simulink model "plltrans"  (R2017a)
settings: Solver=FixedStepAuto  StartTime=0.0  StopTime=150E-6  RelTol=1e-3
libraries: cstblocks x2, simulink x1, hdlsllib x1
settings Model: Creator=fritz  LastModifiedBy=beckmanf
settings OptimizationCC: BlockReduction=off  ConditionallyExecuteInputs=off  DefaultParameterBehavior=Inlined
settings DebuggingCC: AlgebraicLoopMsg=error  SingleTaskRateTransMsg=error
settings HardwareCC: ProdBitPerPointer=32  ProdBitPerSizeT=32  ProdBitPerPtrDiffT=32  ProdLargestAtomicFloat=None  ProdIntDivRoundTo=Undefined  ProdEndianess=Unspecified  ProdWordSize=32  ProdHWDeviceType=ASIC/FPGA->ASIC/FPGA  ProdEqTarget=off

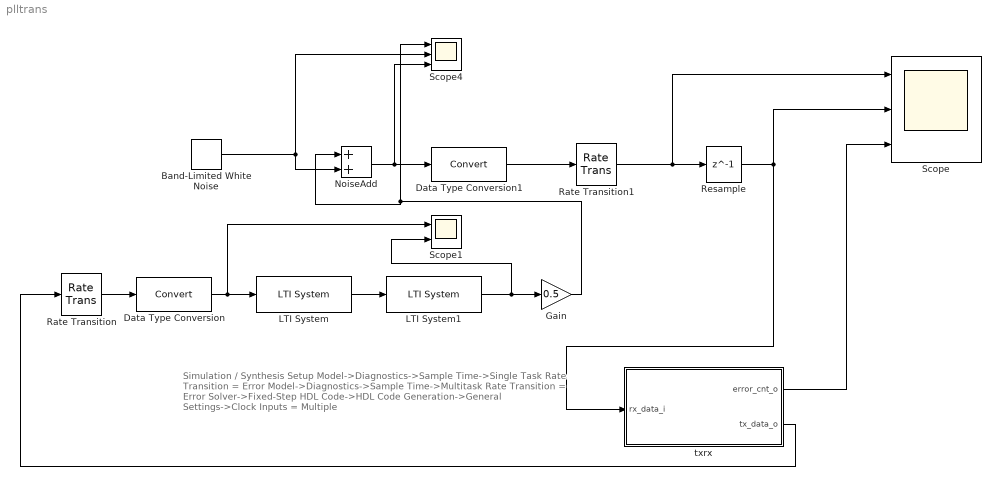
== system plltrans ==
  note: Simulation / Synthesis Setup
      | Model->Diagnostics->Sample Time->Single Task Rate Transition = Error
      | Model->Diagnostics->Sample Time->Multitask Rate Transition = Error
      | Solver->Fixed-Step
      | HDL Code->HDL Code Generation->General Settings->Clock Inputs = Multiple
  Band-Limited White Noise : simulink/Sources/Band-Limited White Noise  Cov=0.05*1/6*1E-9  Ts=1E-9  seed=[23341]
  Data Type Conversion : DataTypeConversion
  Data Type Conversion1 : DataTypeConversion  SaturateOnIntegerOverflow=on
  Gain : Gain  Gain=0.5
  LTI System : cstblocks/LTI System  sys=tf([1 0],[1 1/3.5E-6])  IC=[]
  LTI System1 : cstblocks/LTI System  sys=tf([1 0],[1 1/3.5E-6])  IC=[]
  NoiseAdd : Sum
  Rate Transition : RateTransition
  Rate Transition1 : RateTransition
  Resample : Delay  DelayLength=1  SampleTime=20E-9
  Scope : Scope  NumInputPorts=3
  Scope1 : Scope  NumInputPorts=2
  Scope4 : Scope  NumInputPorts=3
  txrx : Subsystem
  wires:
  Band-Limited White Noise/1 -> NoiseAdd/2, Scope4/2
  NoiseAdd/1 -> Data Type Conversion1/1, Scope4/3
  Resample/1 -> txrx/1(rx_data_i), Scope/2
  Data Type Conversion/1 -> LTI System/1, Scope1/1
  Gain/1 -> Scope4/1, NoiseAdd/1
  txrx/1(error_cnt_o) -> Scope/3
  txrx/2(tx_data_o) -> Rate Transition/1
  Rate Transition/1 -> Data Type Conversion/1
  Data Type Conversion1/1 -> Rate Transition1/1
  Rate Transition1/1 -> Resample/1, Scope/1
  LTI System/1 -> LTI System1/1
  LTI System1/1 -> Scope1/2, Gain/1

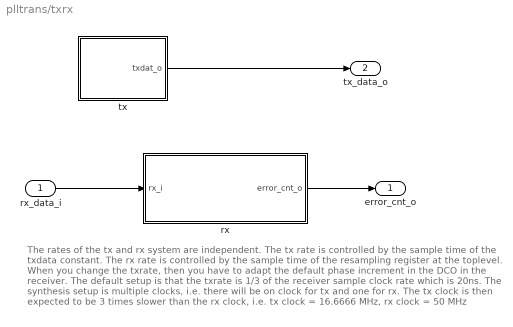
== system plltrans/txrx ==
  note: The rates of the tx and rx system are independent. The tx rate is controlled by the sample time of the
      | txdata constant. The rx rate is controlled by the sample time of the resampling register at the toplevel.
      | When you change the txrate, then you have to adapt the default phase increment in the DCO in the receiver.
      | The default setup is that the txrate is 1/3 of the receiver sample clock rate which is 20ns. The
      | synthesis setup is multiple clocks, i.e. there will be on clock for tx and one for rx. The tx clock is then
      | expected to be 3 times slower than the rx clock, i.e. tx clock = 16.6666 MHz, rx clock = 50 MHz
  rx_data_i : Inport  OutDataTypeStr=fixdt(1,14,13)
  rx : Subsystem
  tx : Subsystem
  error_cnt_o : Outport  OutDataTypeStr=fixdt(0,10,0)
  tx_data_o : Outport  Port=2  OutDataTypeStr=fixdt(1,14,13)
  wires:
  tx/1(txdat_o) -> tx_data_o/1
  rx/1(error_cnt_o) -> error_cnt_o/1
  rx_data_i/1 -> rx/1(rx_i)

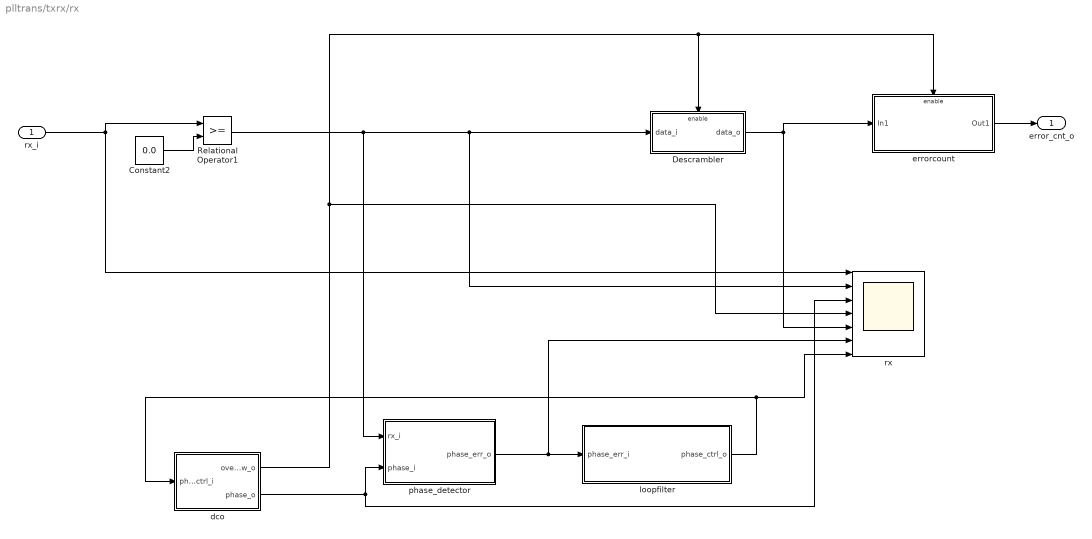
== system plltrans/txrx/rx ==
  rx_i : Inport  OutDataTypeStr=fixdt(1,14,13)
  Constant2 : Constant  Value=0.0  OutDataTypeStr=Inherit: Inherit via back propagation
  Descrambler : Subsystem  TreatAsAtomicUnit=on
  Relational Operator1 : RelationalOperator  OutDataTypeStr=boolean  RndMeth=Nearest
  dco : Subsystem
  errorcount : Subsystem
  loopfilter : Subsystem
  phase_detector : Subsystem
  rx : Scope  NumInputPorts=7
  error_cnt_o : Outport
  wires:
  rx_i/1 -> rx/1, Relational Operator1/1
  phase_detector/1(phase_err_o) -> rx/6, loopfilter/1(phase_err_i)
  loopfilter/1(phase_ctrl_o) -> rx/7, dco/1(phase_ctrl_i)
  dco/2(phase_o) -> phase_detector/2(phase_i), rx/3
  Constant2/1 -> Relational Operator1/2
  Descrambler/1(data_o) -> errorcount/1(In1), rx/5
  Relational Operator1/1 -> rx/2, Descrambler/1(data_i), phase_detector/1(rx_i)
  errorcount/1(Out1) -> error_cnt_o/1
  dco/1(overflow_o) -> errorcount/Enable, Descrambler/Enable, rx/4

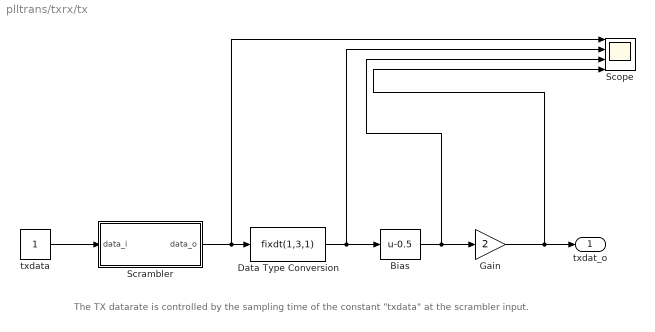
== system plltrans/txrx/tx ==
  note: The TX datarate is controlled by the sampling time of the constant "txdata" at the scrambler input.
  Bias : Bias  Bias=-0.5
  Data Type Conversion : DataTypeConversion  OutDataTypeStr=fixdt(1,3,1)  RndMeth=Nearest
  Gain : Gain  Gain=2  OutDataTypeStr=Inherit: Inherit via back propagation  SaturateOnIntegerOverflow=on
  Scope : Scope  NumInputPorts=4
  Scrambler : Subsystem  TreatAsAtomicUnit=on
  txdata : Constant  OutDataTypeStr=Inherit: Inherit via back propagation  SampleTime=60E-9
  txdat_o : Outport  OutDataTypeStr=fixdt(1,14,13)
  wires:
  txdata/1 -> Scrambler/1(data_i)
  Bias/1 -> Scope/3, Gain/1
  Gain/1 -> Scope/4, txdat_o/1
  Scrambler/1(data_o) -> Scope/1, Data Type Conversion/1
  Data Type Conversion/1 -> Scope/2, Bias/1

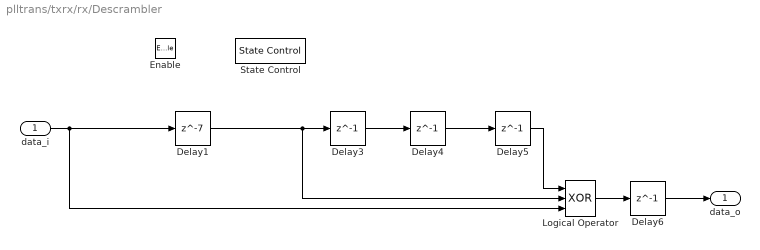
== system plltrans/txrx/rx/Descrambler ==
  data_i : Inport
  Enable : EnablePort
  Delay1 : Delay  DelayLength=7  InitialCondition=0
  Delay{3..6} (4 alike) : Delay  DelayLength=1  InitialCondition=0
  Logical Operator : Logic  Operator=XOR  Inputs=3  AllPortsSameDT=off  OutDataTypeStr=boolean
  State Control : StateControl  StateControl=Synchronous
  data_o : Outport
  wires:
  data_i/1 -> Delay1/1, Logical Operator/3
  Delay4/1 -> Delay5/1
  Delay3/1 -> Delay4/1
  Delay1/1 -> Logical Operator/2, Delay3/1
  Delay5/1 -> Logical Operator/1
  Logical Operator/1 -> Delay6/1
  Delay6/1 -> data_o/1

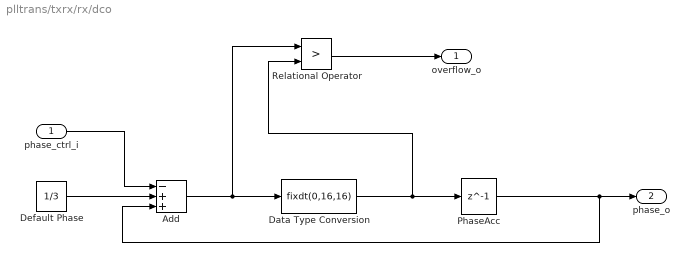
== system plltrans/txrx/rx/dco ==
  phase_ctrl_i : Inport
  Add : Sum  Inputs=-++  AccumDataTypeStr=fixdt(0,18,16)
  Data Type Conversion : DataTypeConversion  OutDataTypeStr=fixdt(0,16,16)  RndMeth=Zero
  Default Phase : Constant  Value=1/3  OutDataTypeStr=Inherit: Inherit via back propagation
  PhaseAcc : Delay  DelayLength=1
  Relational Operator : RelationalOperator  Operator=>  OutDataTypeStr=boolean  ZeroCross=off  RndMeth=Nearest
  overflow_o : Outport
  phase_o : Outport  Port=2
  wires:
  Default Phase/1 -> Add/2
  PhaseAcc/1 -> phase_o/1, Add/3
  Relational Operator/1 -> overflow_o/1
  Add/1 -> Relational Operator/1, Data Type Conversion/1
  Data Type Conversion/1 -> PhaseAcc/1, Relational Operator/2
  phase_ctrl_i/1 -> Add/1

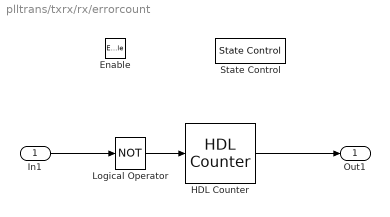
== system plltrans/txrx/rx/errorcount ==
  In1 : Inport
  Enable : EnablePort
  HDL Counter : hdlsllib/HDL Operations/HDL Counter  CountType=Count limited  CountInit=0  CountStep=1  CountMax=1023  CountFromType=Specify  CountFrom=0  CountResetPort=off  CountLoadPort=off  CountEnbPort=on  CountDirPort=off  CountDataType=Unsigned  CountWordLen=10  CountFracLen=0  CountSampTime=1
      settings: SourceProductName=HDL Coder  SourceProductBaseCode=HD
  Logical Operator : Logic  Operator=NOT  AllPortsSameDT=off  OutDataTypeStr=boolean
  State Control : StateControl  StateControl=Synchronous
  Out1 : Outport
  wires:
  Logical Operator/1 -> HDL Counter/1
  HDL Counter/1 -> Out1/1
  In1/1 -> Logical Operator/1

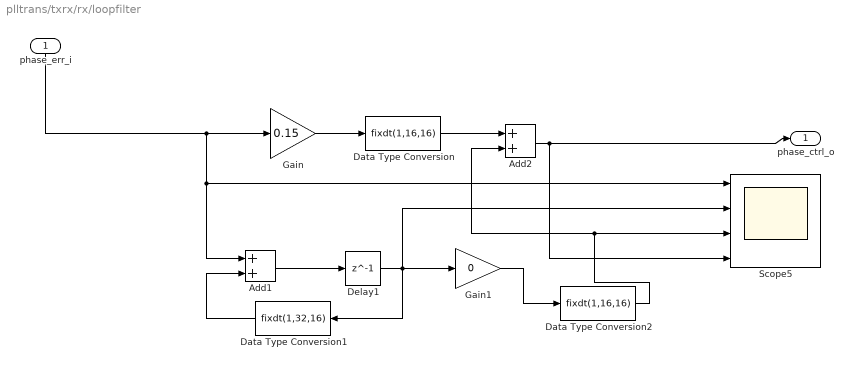
== system plltrans/txrx/rx/loopfilter ==
  phase_err_i : Inport
  Add1 : Sum  AccumDataTypeStr=fixdt(1,32,16)
  Add2 : Sum
  Data Type Conversion : DataTypeConversion  OutDataTypeStr=fixdt(1,16,16)
  Data Type Conversion1 : DataTypeConversion  OutDataTypeStr=fixdt(1,32,16)
  Data Type Conversion2 : DataTypeConversion  OutDataTypeStr=fixdt(1,16,16)
  Delay1 : Delay  DelayLength=1
  Gain : Gain  Gain=0.15
  Gain1 : Gain  Gain=0
  Scope5 : Scope  NumInputPorts=4
  phase_ctrl_o : Outport
  wires:
  phase_err_i/1 -> Gain/1, Scope5/1, Add1/1
  Delay1/1 -> Data Type Conversion1/1, Gain1/1, Scope5/2
  Add1/1 -> Delay1/1
  Gain1/1 -> Data Type Conversion2/1
  Add2/1 -> phase_ctrl_o/1, Scope5/4
  Gain/1 -> Data Type Conversion/1
  Data Type Conversion/1 -> Add2/1
  Data Type Conversion1/1 -> Add1/2
  Data Type Conversion2/1 -> Add2/2, Scope5/3

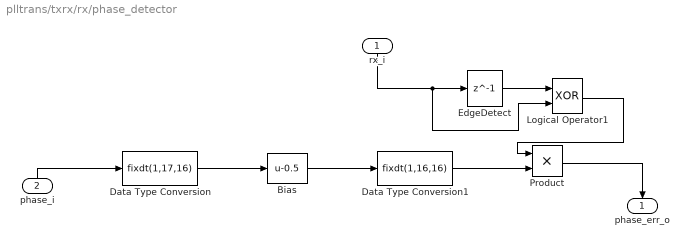
== system plltrans/txrx/rx/phase_detector ==
  rx_i : Inport
  phase_i : Inport  Port=2
  Bias : Bias  Bias=-0.5
  Data Type Conversion : DataTypeConversion  OutDataTypeStr=fixdt(1,17,16)
  Data Type Conversion1 : DataTypeConversion  OutDataTypeStr=fixdt(1,16,16)
  EdgeDetect : Delay  DelayLength=1
  Logical Operator1 : Logic  Operator=XOR  AllPortsSameDT=off  OutDataTypeStr=boolean
  Product : Product
  phase_err_o : Outport
  wires:
  phase_i/1 -> Data Type Conversion/1
  rx_i/1 -> EdgeDetect/1, Logical Operator1/2
  Bias/1 -> Data Type Conversion1/1
  EdgeDetect/1 -> Logical Operator1/1
  Logical Operator1/1 -> Product/1
  Product/1 -> phase_err_o/1
  Data Type Conversion/1 -> Bias/1
  Data Type Conversion1/1 -> Product/2

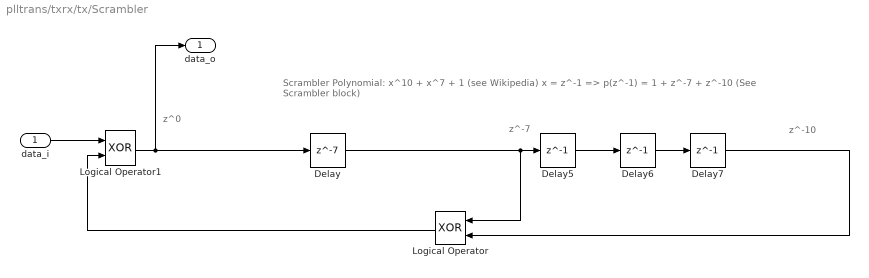
== system plltrans/txrx/tx/Scrambler ==
  note: z^-10
  note: Scrambler Polynomial: x^10 + x^7 + 1 (see Wikipedia) x = z^-1 => p(z^-1) = 1 + z^-7 + z^-10 (See Scrambler block)
  note: z^-7
  note: z^0
  data_i : Inport
  Delay : Delay  DelayLength=7  InitialCondition=0
  Delay5 : Delay  DelayLength=1  InitialCondition=0
  Delay6 : Delay  DelayLength=1  InitialCondition=0
  Delay7 : Delay  DelayLength=1  InitialCondition=0
  Logical Operator : Logic  Operator=XOR  AllPortsSameDT=off  OutDataTypeStr=boolean
  Logical Operator1 : Logic  Operator=XOR  AllPortsSameDT=off  OutDataTypeStr=boolean
  data_o : Outport
  wires:
  Delay/1 -> Logical Operator/1, Delay5/1
  Logical Operator/1 -> Logical Operator1/2
  Logical Operator1/1 -> data_o/1, Delay/1
  data_i/1 -> Logical Operator1/1
  Delay7/1 -> Logical Operator/2
  Delay5/1 -> Delay6/1
  Delay6/1 -> Delay7/1
